simulink model "MySimulationModel"  (R2024b)
settings: Solver=VariableStepAuto  StartTime=0.0  StopTime=10.0  RelTol=1e-3
undefined symbols (not defined in the file): DiscIntNeverNeededParam
settings Model: Creator=xinxing  LastModifiedBy=xinxing

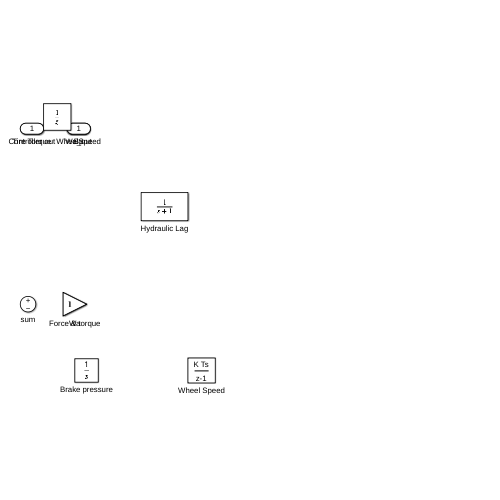
[thumbnail: Simulink's stored preview of the top-level diagram]
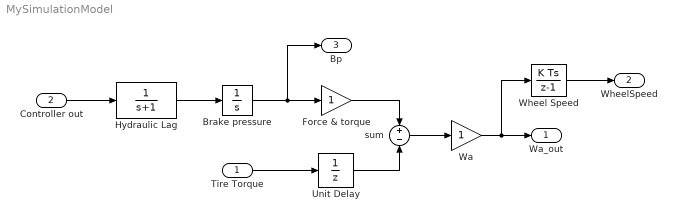
== system MySimulationModel ==
  Tire Torque : Inport
  Controller out : Inport  Port=2
  Brake pressure : Integrator
  Force & torque : Gain
  Hydraulic Lag : TransferFcn  Denominator=[1 1]
  Unit Delay : UnitDelay  SampleTime=-1  HasFrameUpgradeWarning=on
  Wa : Gain
  Wheel Speed : DiscreteIntegrator  SampleTime=-1  ICPrevOutput=DiscIntNeverNeededParam  ICPrevScaledInput=DiscIntNeverNeededParam
  sum : Sum  Inputs=+-
  Wa_out : Outport
  WheelSpeed : Outport  Port=2
  Bp : Outport  Port=3
  wires:
  Wheel Speed/1 -> WheelSpeed/1
  Wa/1 -> Wa_out/1, Wheel Speed/1
  sum/1 -> Wa/1
  Tire Torque/1 -> Unit Delay/1
  Force & torque/1 -> sum/1
  Brake pressure/1 -> Bp/1, Force & torque/1
  Unit Delay/1 -> sum/2
  Hydraulic Lag/1 -> Brake pressure/1
  Controller out/1 -> Hydraulic Lag/1
